simulink model "simulink_example1"  (Simulink 7.1)
settings: Solver=ode45  StartTime=0.0  StopTime=2  RelTol=1e-3
undefined symbols (not defined in the file): a, K1, Kp
settings Model: Creator=ahp  LastModifiedBy=ahp

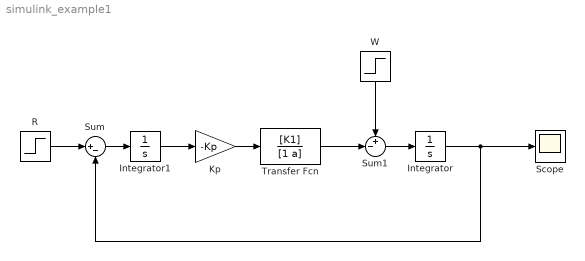
== system simulink_example1 ==
  Integrator : Integrator
  Integrator1 : Integrator
  Kp : Gain  Gain=-Kp  ParameterDataType=sfix(16)  ParameterScaling=2^0  OutDataType=sfix(16)  OutScaling=2^0
  R : Step  SampleTime=0
  Scope : Scope
  Sum : Sum  Inputs=|+-  OutDataType=sfix(16)  OutScaling=2^0
  Sum1 : Sum  Inputs=+-|  OutDataType=sfix(16)  OutScaling=2^0
  Transfer Fcn : TransferFcn  Numerator=[K1]  Denominator=[1 a]
  W : Step  Orientation=down  Time=5  SampleTime=0
  wires:
  R/1 -> Sum/1
  Sum/1 -> Integrator1/1
  Kp/1 -> Transfer Fcn/1
  Transfer Fcn/1 -> Sum1/2
  W/1 -> Sum1/1
  Sum1/1 -> Integrator/1
  Integrator/1 -> Scope/1, Sum/2
  Integrator1/1 -> Kp/1
